simulink model "New_Energy_Model_2"  (R2019a)
settings: Solver=VariableStepAuto  StartTime=0.0  StopTime=834  RelTol=1e-3
libraries: ee_lib x3, powerlib x2, electricdrivelib x1
settings Model: Creator=eabrowning  LastModifiedBy=eabrowning

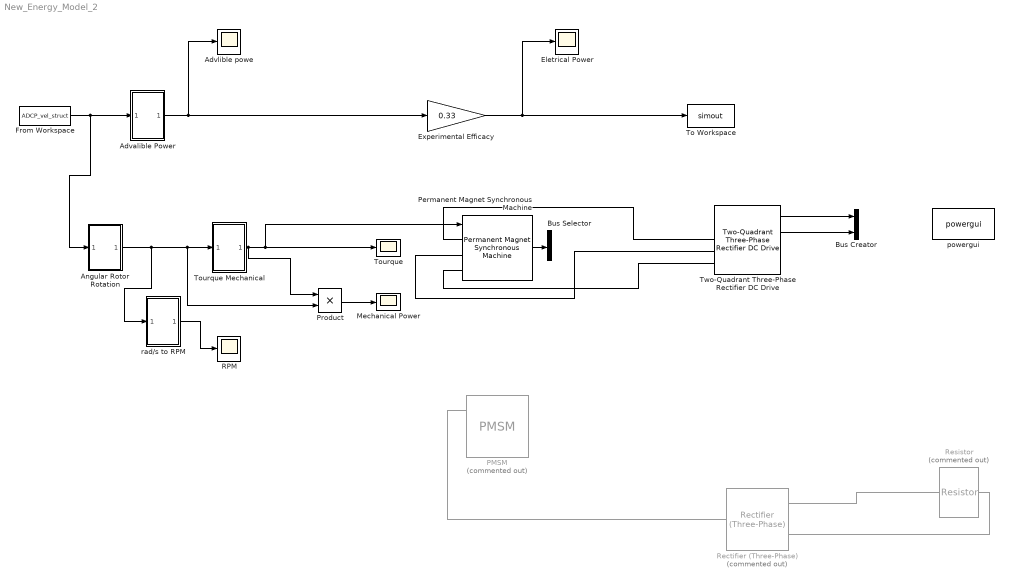
== system New_Energy_Model_2 ==
  " Tourque Mechanical" : Subsystem
  Advalible Power : Subsystem
  "Advlible powe " : Scope
  Angular Rotor Rotation : Subsystem
  Bus Creator : BusCreator  Inputs=2
  Bus Selector : BusSelector  OutputSignals=vqs,vds,ias,ibs,ics,iqs
  "Eletrical Power " : Scope
  Experimental Efficacy : Gain  Gain=0.33
  From Workspace : FromWorkspace  VariableName=ADCP_vel_struct  OutDataTypeStr=double  SampleTime=2  OutputAfterFinalValue=Holding final value
  Mechanical Power : Scope
  PMSM : ee_lib/Electromechanical/Permanent Magnet/PMSM  Commented=on  nPolePairs=6  pmflux_param=1  pm_flux_linkage=0.03 Wb  torque_constant=0.18 N*m/A  back_emf_constant=0.18 V/(rad/s)  stator_param=1  Ld=0.00019 H  Lq=0.00025 H  L0=0.00016 H  Ls=0.0002 H  Lm=-0.00002 H  Ms=0.00002 H  Rs=0.013 Ohm  zero_sequence=ee.enum.park.zerosequence.include  J=0.01 kg*m^2  lam=0 N*m/(rad/s)  axes_param=ee.enum.rotorangle.daxis  i_d_specify=off  i_d_priority=None  i_d=0 A  i_d_nominal_specify=off  i_d_nominal_unit=A  i_d_nominal_value=1  i_q_specify=off  i_q_priority=None  i_q=0 A  i_q_nominal_specify=off  i_q_nominal_unit=A  i_q_nominal_value=1  torque_specify=off  torque_priority=None  torque=0 N*m  torque_nominal_specify=off  torque_nominal_unit=N*m  torque_nominal_value=1  angular_velocity_specify=off  angular_velocity_priority=High  angular_velocity=0 rpm  angular_velocity_nominal_specify=off  angular_velocity_nominal_unit=rpm  angular_velocity_nominal_value=1  angular_position_specify=off  angular_position_priority=High  angular_position=0 deg  angular_position_nominal_specify=off  angular_position_nominal_unit=deg  angular_position_nominal_value=1
      settings: SourceProductName=Simscape Electrical
  Permanent Magnet Synchronous Machine : powerlib/Machines/Permanent Magnet Synchronous Machine  NbPhases=3  FluxDistribution=Sinusoidal  RotorType=Round  MechanicalLoad=Torque Tm  PresetModel=No  ShowDetailedParameters=on  MeasurementBus=on  Resistance=0.4578  Inductance=8.5e-3  dqInductances=[8.5e-3,8.5e-3]  La=0.00334  MachineConstant=Flux linkage established by magnets (V.s)  Flux=0.171  VoltageCst=124.0639  TorqueCst=1.026  Flat=120  Mechanical=[0.001469 0.0003035 4 0]  PolePairs=4  InitialConditions=[0,0, 0,0]  InitialConditions5ph=[0 0 0 0 0 0]  TsPowergui=0  TsBlock=-1  RefAngle=90 degrees behind phase A axis (modified Park)
  Product : Product
  RPM : Scope
  Rectifier (Three-Phase) : ee_lib/Semiconductors & Converters/Converters/Rectifier (Three-Phase)  Commented=on  model_dynamics=0  Vf=0.8 V  Ron=0.001 Ohm  Goff=1e-5 1/Ohm  C=50 nF  iRM=-235 A  iF=300 A  idot=-50 A/us  trr_param=1  trr_factor=3  trr=15 us  Qrr=1500 s*uA
      settings: SourceProductName=Simscape Electrical  SourceProductBaseCode=PS
  Resistor : ee_lib/Passive/Resistor  Commented=on  R=20 Ohm  R_tol=5  enable_R_tol=0  tol_distribution=1  nSigma=4  enable_operating_limits=0  operating_limit_action=2  max_working_voltage=100 V  power_rating=1 W  enable_faults=0  fault_action=1  R_faulted=inf Ohm  enable_temporal_fault=0  t_fault=1 s  enable_behavioral_fault=0  max_permissible_current=1 A  t_fail_on_current=1 s  noise_mode=0  sample_time=1e-3 s  repeatability=1  auto_seed=3762145728  user_seed=0  Tdevice=25 degC  alpha=3.93e-3 1/K  Tmeas=25 degC  thermal_mass=100 J/K  power_derating_T1=70 degC  power_derating_T2=155 degC  operating_temperature_range_vec=[-50, 150] degC  temperature_specify=off  temperature_priority=High  temperature=298.15 K  temperature_nominal_specify=off  temperature_nominal_unit=K  temperature_nominal_value=1
      settings: SourceProductName=Simscape Electrical
  To Workspace : ToWorkspace  VariableName=simout  SaveFormat=Timeseries  SampleTime=-1
  Tourque : Scope
  Two-Quadrant Three-Phase Rectifier DC Drive : electricdrivelib/DC drives/Two-Quadrant Three-Phase Rectifier DC Drive  Laf=2.621  Ra=0.0597  La=0.0009  Rf=20  Lf=112.5  J=10  Bm=0.272  Tfriction=0  w0=0  Ron_rec=1e-3  Vf_rec=1.3  Rsnb_rec=4e3  Csnb_rec=900e-9  smoothingInductance=15e-3  Vfield=150  LineVoltage=220  LineFrequency=50  sourceInductance=1e-6  PhaseAngle=0  regulationType=Torque regulation  Tc=100e-6  wb=1750  InitialSpeed=0  fc_sc=40  kp_sc=80  ki_sc=200  Acc=250  Dec=-250  fc_ic=100  refLim=1.5  Pb=200*746  Vb=500  kp_ic=1.5  ki_ic=60  alphamin=20  alphamax=160  freqSynchro=60  pulseWitdth=10  baseSampleTime=5e-05  outputBusMode=Multiple output buses  busLabels=off  MechanicalLoad=Torque Tm  modelDetailLevel=Detailed  driveType=DC3  AverageValue=off
      settings: SourceProductName=Simscape Electrical  SourceProductBaseCode=PS
  powergui : powerlib/powergui  Priority=1  SimulationMode=Discrete  SampleTime=50e-6  frequency=60  Iterations=50  frequencyindice=0  Pbase=100e6  ErrMax=1e-4  UnitsV=kV  UnitsW=MW  buscounter=0  FunctionMessages=off  echomessages=off  EnableUseOfTLC=off  CurrentSourceSwitches=off  DisableSnubberDevices=off  DisableRonSwitches=off  DisableVfSwitches=off  DisplayEquations=off  AutomaticDiscreteSolvers=off  SolverType=Tustin/Backward Euler (TBE)  Interpol=off  ExternalGateDelay=off  methode=off  Ts=100  x0status=blocks  SPID=on  SwTol=0  HookPort=off  NonlinearTolerance=0  nMaxIteration=15  ContinueOnMaxIteration=off  RestoreLinks=warning  ResistiveCurrentMeasurement=off  Frange=[0:2:500]  Ylog=off  Xlog=on  ShowGrid=off  save=off  variable=ZData  structure=0  ZoomFFT=off  StartTime=0.0  cycles=1  DisplayStyle=1  fundamental=60  FreqAxis=off  MaxFrequency=1000  frequencyindicesteady=1  RmsSteady=1  display=off
      settings: SourceProductName=Simscape Electrical
  rad/s to RPM : Subsystem
  wires:
  Experimental Efficacy/1 -> To Workspace/1, "Eletrical Power "/1
  Advalible Power/1(Out1) -> Experimental Efficacy/1, "Advlible powe "/1
  From Workspace/1 -> Angular Rotor Rotation/1(In1), Advalible Power/1(In1)
  Angular Rotor Rotation/1(Out1) -> rad/s to RPM/1(In1), Product/2, " Tourque Mechanical"/1(In1)
  " Tourque Mechanical"/1(Out1) -> Permanent Magnet Synchronous Machine/1, Tourque/1, Product/1
  rad/s to RPM/1(Out1) -> RPM/1
  Product/1 -> Mechanical Power/1
  Permanent Magnet Synchronous Machine/1 -> Bus Selector/1
  Two-Quadrant Three-Phase Rectifier DC Drive/2 -> Bus Creator/2
  Two-Quadrant Three-Phase Rectifier DC Drive/1 -> Bus Creator/1
  connections:
  Rectifier (Three-Phase)/RConn2 -- Resistor/RConn1
  Rectifier (Three-Phase)/RConn1 -- Resistor/LConn1
  PMSM/LConn1 -- Rectifier (Three-Phase)/LConn1
  Permanent Magnet Synchronous Machine/LConn3 -- Two-Quadrant Three-Phase Rectifier DC Drive/LConn3
  Permanent Magnet Synchronous Machine/LConn2 -- Two-Quadrant Three-Phase Rectifier DC Drive/LConn2
  Permanent Magnet Synchronous Machine/LConn1 -- Two-Quadrant Three-Phase Rectifier DC Drive/LConn1

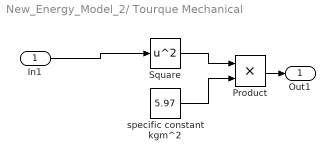
== system New_Energy_Model_2/ Tourque Mechanical ==
  In1 : Inport
  Product : Product
  Square : Math  Operator=square  SaturateOnIntegerOverflow=on
  specific constant kgm^2 : Constant  Value=5.97
  Out1 : Outport
  wires:
  In1/1 -> Square/1
  Square/1 -> Product/1
  specific constant kgm^2/1 -> Product/2
  Product/1 -> Out1/1

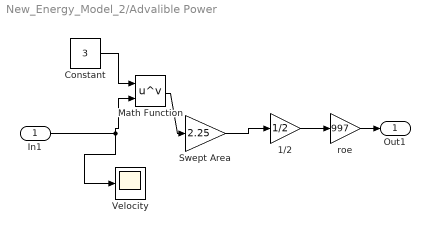
== system New_Energy_Model_2/Advalible Power ==
  In1 : Inport
  1/2 : Gain  Gain=1/2
  Constant : Constant  Value=3
  Math Function : Math  Operator=pow  SaturateOnIntegerOverflow=on
  Swept Area : Gain  Gain=2.25
  Velocity : Scope
  roe : Gain  Gain=997
  Out1 : Outport
  wires:
  Swept Area/1 -> 1/2/1
  In1/1 -> Math Function/2, Velocity/1
  Math Function/1 -> Swept Area/1
  1/2/1 -> roe/1
  Constant/1 -> Math Function/1
  roe/1 -> Out1/1

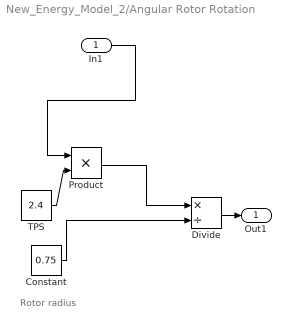
== system New_Energy_Model_2/Angular Rotor Rotation ==
  note: Rotor radius
  In1 : Inport
  Constant : Constant  Value=0.75
  Divide : Product  Inputs=*/
  Product : Product
  "TPS " : Constant  Value=2.4
  Out1 : Outport
  wires:
  Constant/1 -> Divide/2
  "TPS "/1 -> Product/2
  In1/1 -> Product/1
  Divide/1 -> Out1/1
  Product/1 -> Divide/1

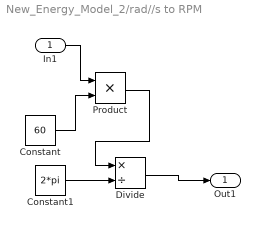
== system New_Energy_Model_2/rad//s to RPM ==
  In1 : Inport
  Constant : Constant  Value=60
  Constant1 : Constant  Value=2*pi
  Divide : Product  Inputs=*/
  Product : Product
  Out1 : Outport
  wires:
  Constant/1 -> Product/2
  Product/1 -> Divide/1
  Divide/1 -> Out1/1
  Constant1/1 -> Divide/2
  In1/1 -> Product/1
